simulink model "CL_"  (R2023a)
settings: Solver=VariableStepAuto  StartTime=0.0  StopTime=Te +Tt -Ts  RelTol=1e-3
values from neighbouring files (symbols this model uses):
  N = 200    [Init.m]    (also in SysIDData_Feedback.mat; motorSystem_Data.mat)
  Ts = 0.002    [Init.m]    (also in SysIDData_Feedback.mat; motorSystem_Data.mat)
  wr = 2*pi/Te    (= 0.418879020479)    [Init.m]    (also in SysIDData_Feedback.mat; motorSystem_Data.mat)
settings Model: Creator=quarc_user  LastModifiedBy=quarc_user

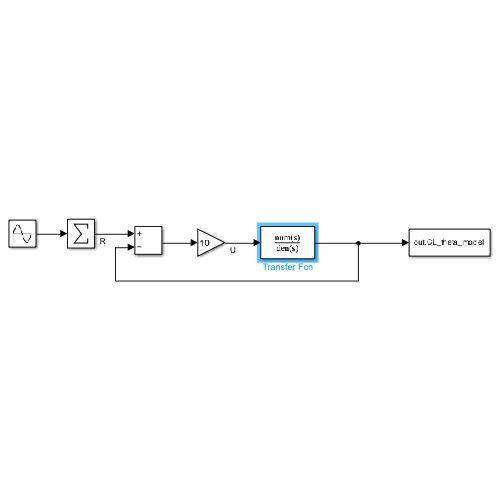
[thumbnail: Simulink's stored preview of the top-level diagram]
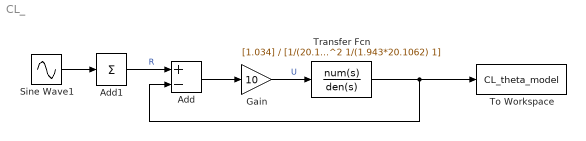
== system CL_ ==
  Add : Sum  Inputs=+-
  Add1 : Sum  Inputs=+
  Gain : Gain  Gain=10
  Sine Wave1 : Sin  Amplitude=0.02  Frequency=[1:N]*wr  Phase=2*pi*rand(1,N)  SampleTime=0
  To Workspace : ToWorkspace  VariableName=CL_theta_model  SampleTime=Ts
      settings: MaxDataPoints=Te/Ts
  Transfer Fcn : TransferFcn  Numerator=[1.034]  Denominator=[1/(20.1062)^2 1/(1.943*20.1062) 1]
  wires:
  Sine Wave1/1 -> Add1/1
  Add1/1 -> Add/1  "R"
  Add/1 -> Gain/1
  Gain/1 -> Transfer Fcn/1  "U"
  Transfer Fcn/1 -> To Workspace/1, Add/2
